simulink model "noise"  (R2025b)
settings: Solver=VariableStepAuto  StartTime=0.0  StopTime=20  RelTol=1e-3
values from neighbouring files (symbols this model uses):
  estim_A = A - B*K - L*C    [integrador.m]    (also in q8.m)
  K = lqr(A, B, Qr, Rr)    [IP_MACRO.m]    (also in Integrador_of_IP_MACRO.m = K_aug(1:5); integrador.m = K_aug(1:5))
  L = lqe(A, G, C, Qe, Re)    [IP_MACRO.m]    (also in Integrador_of_IP_MACRO.m; integrador.m; q7.m; q8.m)
  x0 = [0.1 0 0 0 0]'    [integrador.m]    (also in q8.m)
undefined symbols (not defined in the file or in its folder): A, B, C, D
libraries: simulink x1
settings Model: Creator=matos  LastModifiedBy=matos

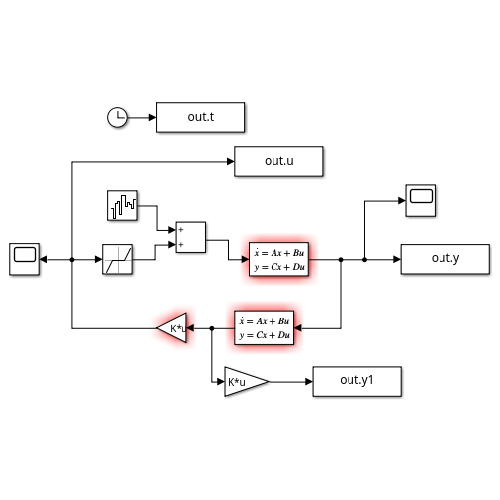
[thumbnail: Simulink's stored preview of the top-level diagram]
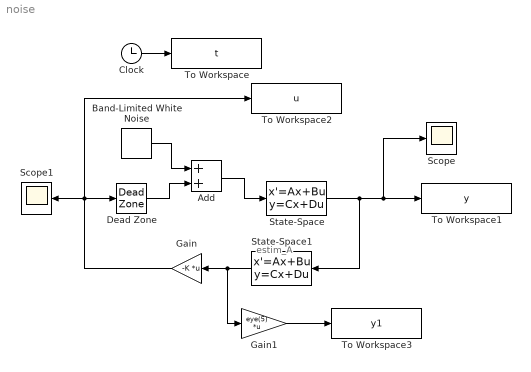
== system noise ==
  note: estim_A
  Add : Sum
  Band-Limited White Noise : simulink/Sources/Band-Limited White Noise  Cov=[0.1]  Ts=0.1  seed=[23341]
  Clock : Clock
  Dead Zone : DeadZone  LowerValue=-0.19  UpperValue=0.19
  Gain : Gain  Gain=-K  Multiplication=Matrix(K*u)
  Gain1 : Gain  Gain=eye(5)  Multiplication=Matrix(K*u)
  Scope : Scope
      settings: ActiveDisplayYMinimum=-0.16877096224018479  ActiveDisplayYMaximum=0.22153069896433672
  Scope1 : Scope
      settings: ActiveDisplayYMinimum=-0.77264121823991716  ActiveDisplayYMaximum=0.76684803695448767
  State-Space : StateSpace  A=A  B=B  C=C  D=D  InitialCondition=x0
  State-Space1 : StateSpace  A=estim_A  B=L  C=eye(5)  D=zeros(5,2)  InitialCondition=0
  To Workspace : ToWorkspace  VariableName=t  SaveFormat=Timeseries  SampleTime=-1
  To Workspace1 : ToWorkspace  VariableName=y  SaveFormat=Timeseries  SampleTime=-1
  To Workspace2 : ToWorkspace  VariableName=u  SaveFormat=Timeseries  SampleTime=-1
  To Workspace3 : ToWorkspace  VariableName=y1  SaveFormat=Timeseries  SampleTime=-1
  wires:
  Clock/1 -> To Workspace/1
  State-Space/1 -> Scope/1, To Workspace1/1, State-Space1/1
  State-Space1/1 -> Gain1/1, Gain/1
  Gain/1 -> Dead Zone/1, To Workspace2/1, Scope1/1
  Gain1/1 -> To Workspace3/1
  Dead Zone/1 -> Add/2
  Band-Limited White Noise/1 -> Add/1
  Add/1 -> State-Space/1
